simulink library "SinglePipe_lib"  (R2019a)
settings: Solver=VariableStepAuto  StartTime=0.0  StopTime=10.0  RelTol=1e-3
settings Model: Creator=martin  LastModifiedBy=martin

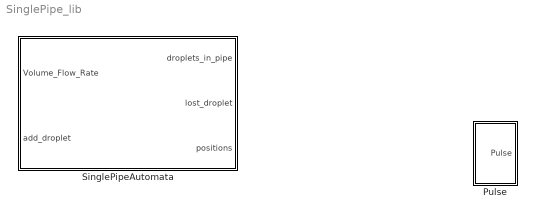
== system SinglePipe_lib ==
  Pulse : Subsystem  mask{time=1, duration=0.01}
      mask prompts: time "Pulse Time"; duration "Pulse Duration"
  SinglePipeAutomata : Subsystem  mask{width=2, length=5, height=3, dt=0.01, R_per_droplet=1}
      mask prompts: width "Pipe Width"; length "Pipe Length"; height "Pipe Height"; dt "time step"; R_per_droplet "Resistance Per Droplet"
      mask TypeOptions dt: Custom_Integrator/dt
      mask TypeOptions R_per_droplet: Custom_Integrator/R_per_droplet

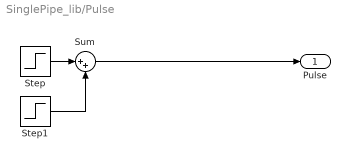
== system SinglePipe_lib/Pulse ==
  Step : Step  Time=time
  Step1 : Step  Time=time+duration  After=-1
  Sum : Sum  Inputs=|++
  Pulse : Outport
  wires:
  Step1/1 -> Sum/2
  Step/1 -> Sum/1
  Sum/1 -> Pulse/1

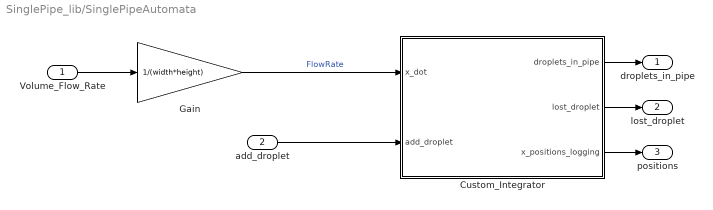
== system SinglePipe_lib/SinglePipeAutomata ==
  Volume_Flow_Rate : Inport
  add_droplet : Inport  Port=2
  Custom_Integrator : MATLAB Function  TreatAsAtomicUnit=on  mask{dt=dt, upper_Limit=length, R_per_droplet=R_per_droplet}
      mask prompts: dt "time step"; upper_Limit "Length of Pipe"; R_per_droplet "Resistance Per Droplet"
  Gain : Gain  Gain=1/(width*height)
  droplets_in_pipe : Outport
  lost_droplet : Outport  Port=2
  positions : Outport  Port=3
  wires:
  Volume_Flow_Rate/1 -> Gain/1
  Gain/1 -> Custom_Integrator/1(x_dot)  "FlowRate"
  add_droplet/1 -> Custom_Integrator/2(add_droplet)
  Custom_Integrator/2(lost_droplet) -> lost_droplet/1
  Custom_Integrator/1(droplets_in_pipe) -> droplets_in_pipe/1
  Custom_Integrator/3(x_positions_logging) -> positions/1

== matlab function SinglePipe_lib/SinglePipeAutomata/Custom_Integrator ==
  data: x_dot input; dt parameter; add_droplet input; upper_Limit parameter; droplets_in_pipe output; R_per_droplet parameter; lost_droplet output; x_positions_logging output size=10
function [droplets_in_pipe, lost_droplet, x_positions_logging] = fcn(x_dot, dt, add_droplet, upper_Limit, R_per_droplet)

%% declare persistent memory/internal state
persistent x_state
persistent number_droplet
%% initalize internal state/memory 
if (isempty(x_state))
    x_state = [];
end
if (isempty(number_droplet))
    number_droplet = 0;
end

%% first check if we added a new droplet to the pipe
if(add_droplet > 0)
    number_droplet = number_droplet+1;
    x_state = [x_state,0];
end

%% now propegate droplet position in pipe
% use first order integration
if (number_droplet>0)
    x_state = x_state + repmat(x_dot, 1, numel(x_state))*dt;
end
%% check if any droplets left the pipe
index = x_state > upper_Limit;
x_state = x_state(~index);
lost_droplet = sum(index);

switch lost_droplet
    case 0
        droplets_in_pipe = number_droplet;
    case 1
        number_droplet = number_droplet - lost_droplet;
        droplets_in_pipe = number_droplet;
    otherwise
        error('out side of valid dynamics, reduce step size to prevent two droplets leaving at the same time')
end

%% Add position output for debug
x_positions_logging = zeros(10,1);

index_log = min([10,number_droplet]);

x_positions_logging(1:index_log) = x_state;
